simulink model "RL_parallelCircuit"  (R2023a)
settings: Solver=VariableStepAuto  StartTime=0.0  StopTime=20.0  RelTol=1e-3
undefined symbols (not defined in the file or in its folder): E, L, R1, R2
settings Model: Creator=kawat  LastModifiedBy=kawat

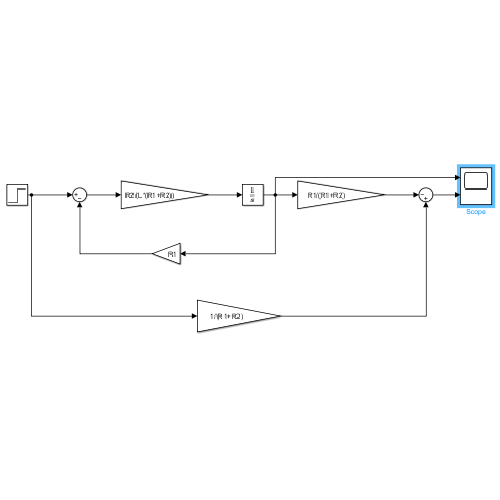
[thumbnail: Simulink's stored preview of the top-level diagram]
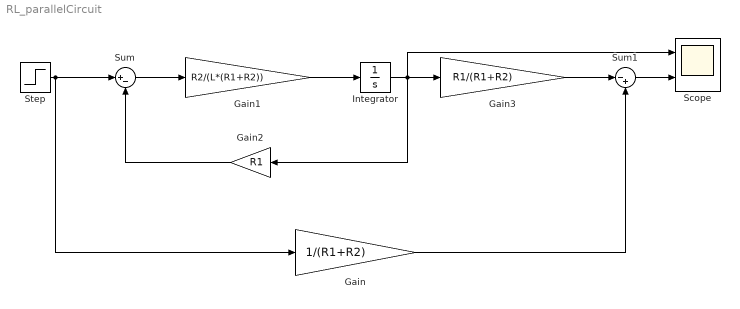
== system RL_parallelCircuit ==
  Gain : Gain  Gain=1/(R1+R2)
  Gain1 : Gain  Gain=R2/(L*(R1+R2))
  Gain2 : Gain  Gain=R1
  Gain3 : Gain  Gain=R1/(R1+R2)
  Integrator : Integrator
  Scope : Scope  NumInputPorts=2
  Step : Step  After=E  SampleTime=0
  Sum : Sum  Inputs=|+-
  Sum1 : Sum  Inputs=|-+
  wires:
  Step/1 -> Gain/1, Sum/1
  Sum/1 -> Gain1/1
  Gain2/1 -> Sum/2
  Gain1/1 -> Integrator/1
  Integrator/1 -> Gain2/1, Gain3/1, Scope/1
  Gain3/1 -> Sum1/1
  Sum1/1 -> Scope/2
  Gain/1 -> Sum1/2
